simulink model "Sensorless_Fault_Tolerant_Control_IM_2"  (R2024a)
settings: Solver=VariableStepAuto  StartTime=0.0  StopTime=2  RelTol=1e-3
values from neighbouring files (symbols this model uses):
  Lm = 0.135    [Step_3_SVPWM.m]    (also in Step_With_MRAS_2c.m = 0.0055; Will_Check_3_Hk_2.m = 0.2)
  Ts = 1e-4    (= 0.0001)    [Step_3_SVPWM.m]    (also in Step_With_MRAS_2c.m; Will_Check_3_Hk_2.m)
undefined symbols (not defined in the file or in its folder): DiscIntNeverNeededParam, Ki, Kp, Param_Limit, R, S, Zp
libraries: spsACVoltageSourceLib x3, slpidlib x3, spsUniversalBridgeLib x3, spsCurrentMeasurementLib x3, spsVoltageMeasurementLib x3, spsAsynchronousMachineSIUnitsLib x2, spsDCVoltageSourceLib x1, spsAlphaBetaZerotodq0Lib x1, spsSVPWMGenerator2LevelLib x1, spsabctoAlphaBetaZeroLib x1, spsdq0toAlphaBetaZeroLib x1, spsGroundLib x1
settings Model: Creator=hkurt  LastModifiedBy=hkurt
settings RTWCC: GPUComputeCapability=3.5

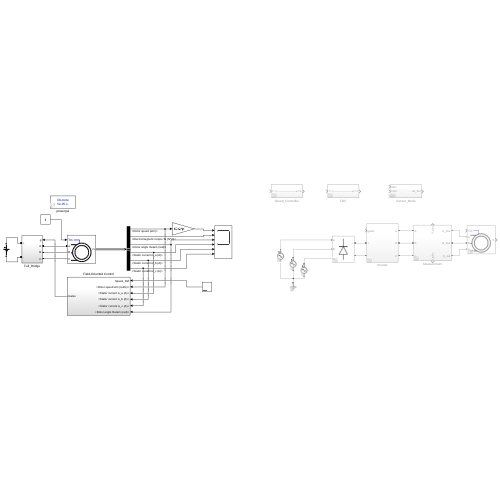
[thumbnail: Simulink's stored preview of the top-level diagram]
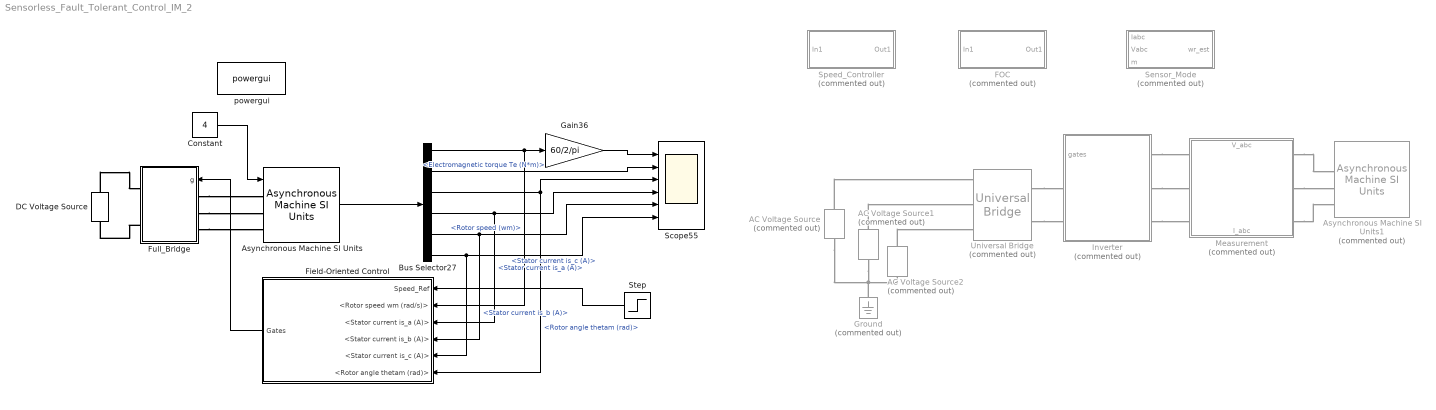
== system Sensorless_Fault_Tolerant_Control_IM_2 ==
  AC Voltage Source : spsACVoltageSourceLib/AC Voltage Source  Commented=on  Amplitude=400/sqrt(3)*sqrt(2)  Phase=0  Frequency=50  SampleTime=0  Measurements=None  BusType=swing  Pref=10e3  Qref=0  Qmin=-inf  Qmax=+inf
  AC Voltage Source1 : spsACVoltageSourceLib/AC Voltage Source  Commented=on  Amplitude=400/sqrt(3)*sqrt(2)  Phase=-120  Frequency=50  SampleTime=0  Measurements=None  BusType=swing  Pref=10e3  Qref=0  Qmin=-inf  Qmax=+inf
  AC Voltage Source2 : spsACVoltageSourceLib/AC Voltage Source  Commented=on  Amplitude=400/sqrt(3)*sqrt(2)  Phase=120  Frequency=50  SampleTime=0  Measurements=None  BusType=swing  Pref=10e3  Qref=0  Qmin=-inf  Qmax=+inf
  Asynchronous Machine SI Units : spsAsynchronousMachineSIUnitsLib/Asynchronous Machine SI Units  RotorType=Squirrel-cage  PresetModel="15:  5.4 HP (4KW)   400 V  50Hz 1430 RPM"  MechanicalLoad=Torque Tm  ShowDetailedParameters=on  ReferenceFrame=Rotor  Units=SI  MeasurementBus=off  NominalParameters=[4000 400 50]  VoltageRatio=1  Stator=[1.405 0.005839]  Rotor=[1.395 0.005839]  Cage1=[0.4155 0.002066]  Cage2=[0.4168 0.0003495]  Lm=0.1722  Mechanical=[0.0131 0.002985 2]  PolePairs=2  InitialConditions=[0 0 0 0 0 0 0 0]  SimulateSaturation=off  Saturation=[14.03593122, 27.81365428, 53.79336849, 72.68890987, 97.98006896, 148.6815601, 215.7428561, 302.9841135, 428.7778367 ; 230, 322, 414, 460, 506, 552, 598, 644, 690]  LoadFlowParameters=1492000  TsPowergui=0  TsBlock=-1  IterativeModel=Trapezoidal non iterative  IterativeDiscreteModel=Trapezoidal non iterative  Pmec=1.492e+006
  Asynchronous Machine SI Units1 : spsAsynchronousMachineSIUnitsLib/Asynchronous Machine SI Units  Commented=on  RotorType=Squirrel-cage  PresetModel="15:  5.4 HP (4KW)   400 V  50Hz 1430 RPM"  MechanicalLoad=Torque Tm  ShowDetailedParameters=on  ReferenceFrame=Rotor  Units=SI  MeasurementBus=off  NominalParameters=[4000 400 50]  VoltageRatio=1  Stator=[1.405 0.005839]  Rotor=[1.395 0.005839]  Cage1=[0.4155 0.002066]  Cage2=[0.4168 0.0003495]  Lm=0.1722  Mechanical=[0.0131 0.002985 2]  PolePairs=2  InitialConditions=[0 0 0 0 0 0 0 0]  SimulateSaturation=off  Saturation=[14.03593122, 27.81365428, 53.79336849, 72.68890987, 97.98006896, 148.6815601, 215.7428561, 302.9841135, 428.7778367 ; 230, 322, 414, 460, 506, 552, 598, 644, 690]  LoadFlowParameters=1492000  TsPowergui=0  TsBlock=-1  IterativeModel=Trapezoidal non iterative  IterativeDiscreteModel=Trapezoidal non iterative  Pmec=1.492e+006
  Bus Selector27 : BusSelector  OutputSignals=Mechanical.Rotor speed (wm),Mechanical.Electromagnetic torque Te (N*m),Mechanical.Rotor angle thetam (rad),Stator measurements.Stator current is_a (A),Stator measurements.Stator current is_b (A),Stator measurements.Stator current is_c (A)
  Constant : Constant  Value=4
  DC Voltage Source : spsDCVoltageSourceLib/DC Voltage Source  Amplitude=690  Measurements=None
  FOC : Subsystem  Commented=on
  Field-Oriented Control : Subsystem
  Full_Bridge : Subsystem
  Gain36 : Gain  Gain=60/2/pi
  Ground : spsGroundLib/Ground  Commented=on  LConnTagsString=a
  Inverter : Subsystem  Commented=on
  Measurement : Subsystem  Commented=on
      settings: PortSchema="{\"entries\":[{\"content\":{\"sides\":[{\"content\":{\"connectorIds\":[\"LConn1\",\"LConn2\",\"LConn3\"]},\"type\":\"ConnectorPlacement.EquallySpacedRectSide\",\"uuid\":\"2eb851a7-a296-4371-9492-5b9a24d98dc4\"},{\"content\":{\"connectorIds\":[\"RConn1\",\"RConn2\",\"RConn3\"],\"side\":\"RIGHT\"},\"type\":\"ConnectorPlacement.EquallySpacedRectSide\",\"uuid\":\"c9fabae8-70a9-40e0-bc91-dae6b4a86947\"},{\"content\":{\"connectorIds\":[\"Out2\"],\"side\":\"TOP\"},\"type\":\"ConnectorPlacement.EquallySpacedRectSide\",\"uuid\":\"f74854e5-c5df-4cc2-afef-707541dbedfe\"},{\"content\":{\"connectorIds\":[\"Out1\"],\"side\":\"BOTTOM\"},\"type\":\"ConnectorPlacement.EquallySpacedRectSide\",\"uuid\":\"696e7b86-8c4f-415d-8e64-0810cecd3876\"}]},\"type\":\"ConnectorPlacement.EquallySpacedConnector\",\"uuid\":\"1b4277bd-9dcb-424e-8124-b504b127c8b4\"}],\"packageUris\":[\"http://schema.mathworks.com/mf0/Connector/R2020b\"],\"version\":\"1.0\"}"
  Scope55 : Scope  NumInputPorts=6
  Sensor_Mode : Subsystem  Commented=on
  Speed_Controller : Subsystem  Commented=on
  Step : Step  Time=0.5  After=1200  SampleTime=0
  Universal Bridge : spsUniversalBridgeLib/Universal Bridge  Commented=on  Arms=3  SnubberResistance=1e5  SnubberCapacitance=inf  Device=Diodes  Ron=1e-3  Lon=0  ForwardVoltages="[  0  0  ]"  ForwardVoltage=0  GTOparameters=[ 10e-6 , 20e-6 ]  IGBTparameters=[ 1e-6 , 2e-6 ]  Measurements=None  Measurements_2=None  converterType=Rectifier
  powergui : sps_lib/powergui  Priority=1  SimulationMode=Discrete  SampleTime=50e-6  frequency=60  Iterations=50  frequencyindice=0  Pbase=100e6  ErrMax=1e-4  UnitsV=kV  UnitsW=MW  buscounter=0  FunctionMessages=off  echomessages=off  EnableUseOfTLC=off  CurrentSourceSwitches=off  DisableSnubberDevices=off  DisableRonSwitches=off  DisableVfSwitches=off  DisplayEquations=off  AutomaticDiscreteSolvers=off  SolverType=Tustin/Backward Euler (TBE)  Interpol=off  ExternalGateDelay=off  methode=off  Ts=100  x0status=blocks  SPID=on  SwTol=0  HookPort=off  NonlinearTolerance=1e-4  nMaxIteration=100  ContinueOnMaxIteration=off  RestoreLinks=warning  ResistiveCurrentMeasurement=off  Frange=[0:2:500]  Ylog=off  Xlog=on  ShowGrid=off  save=off  variable=ZData  structure=0  ZoomFFT=off  StartTime=0.0  cycles=1  DisplayStyle=1  fundamental=60  FreqAxis=off  MaxFrequency=1000  frequencyindicesteady=1  RmsSteady=1  display=off
  wires:
  Field-Oriented Control/1(Gates) -> Full_Bridge/1(g)
  Asynchronous Machine SI Units/1 -> Bus Selector27/1
  Gain36/1 -> Scope55/1
  Bus Selector27/1 -> Gain36/1, Field-Oriented Control/2(<Rotor speed wm (rad/s)>)  "<Rotor speed (wm)>"
  Bus Selector27/2 -> Scope55/2  "<Electromagnetic torque Te (N*m)>"
  Bus Selector27/3 -> Field-Oriented Control/6(<Rotor angle thetam (rad)>), Scope55/3  "<Rotor angle thetam (rad)>"
  Bus Selector27/4 -> Scope55/4, Field-Oriented Control/3(<Stator current is_a (A)>)  "<Stator current is_a (A)>"
  Bus Selector27/5 -> Field-Oriented Control/4(<Stator current is_b (A)>), Scope55/5  "<Stator current is_b (A)>"
  Bus Selector27/6 -> Scope55/6, Field-Oriented Control/5(<Stator current is_c (A)>)  "<Stator current is_c (A)>"
  Constant/1 -> Asynchronous Machine SI Units/1
  Step/1 -> Field-Oriented Control/1(Speed_Ref)
  connections:
  Full_Bridge/LConn1 -- Asynchronous Machine SI Units/LConn1
  Full_Bridge/LConn2 -- Asynchronous Machine SI Units/LConn2
  Full_Bridge/LConn3 -- Asynchronous Machine SI Units/LConn3
  DC Voltage Source/RConn1 -- Full_Bridge/RConn1
  Full_Bridge/RConn2 -- DC Voltage Source/LConn1
  Measurement/RConn1 -- Asynchronous Machine SI Units1/LConn1
  Measurement/RConn2 -- Asynchronous Machine SI Units1/LConn2
  Measurement/RConn3 -- Asynchronous Machine SI Units1/LConn3
  Inverter/RConn1 -- Measurement/LConn1
  Inverter/RConn2 -- Measurement/LConn2
  Inverter/RConn3 -- Measurement/LConn3
  Universal Bridge/RConn1 -- Inverter/LConn1
  Universal Bridge/RConn2 -- Inverter/LConn2
  AC Voltage Source/RConn1 -- Universal Bridge/LConn1
  AC Voltage Source1/RConn1 -- Universal Bridge/LConn2
  AC Voltage Source2/RConn1 -- Universal Bridge/LConn3
  Ground/LConn1 -- AC Voltage Source1/LConn1 -- AC Voltage Source/LConn1 -- AC Voltage Source2/LConn1

== system Sensorless_Fault_Tolerant_Control_IM_2/FOC ==
  In1 : Inport
  Out1 : Outport
  wires:
  In1/1 -> Out1/1

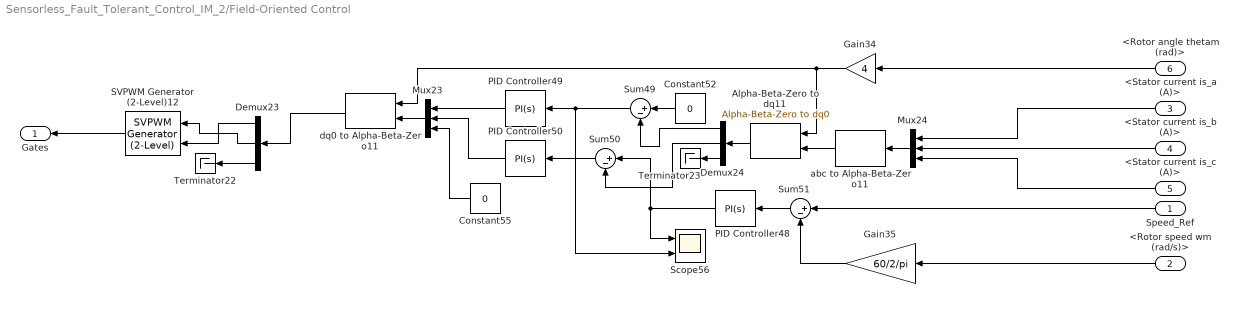
== system Sensorless_Fault_Tolerant_Control_IM_2/Field-Oriented Control ==
  Speed_Ref : Inport
  <Rotor speed wm (rad/s)> : Inport  Port=2
  <Stator current is_a (A)> : Inport  Port=3
  <Stator current is_b (A)> : Inport  Port=4
  <Stator current is_c (A)> : Inport  Port=5
  <Rotor angle thetam (rad)> : Inport  Port=6
  Alpha-Beta-Zero to dq11 : spsAlphaBetaZerotodq0Lib/Alpha-Beta-Zero to dq0  Alignment=90 degrees behind phase A axis
  Constant52 : Constant  Value=0
  Constant55 : Constant  Value=0
  Demux23 : Demux  Outputs=3
  Demux24 : Demux  Outputs=3
  Gain34 : Gain  Gain=4
  Gain35 : Gain  Gain=60/2/pi
  Mux23 : Mux  Inputs=3
  Mux24 : Mux  Inputs=3
  PID Controller48 : slpidlib/PID Controller  Controller=PI  Form=Parallel  TimeDomain=Continuous-time  UseExternalTs=off  SampleTime=-1  IntegratorMethod=Forward Euler  FilterMethod=Forward Euler  ControllerParametersSource=internal  P=0.5  I=10  UseKiTs=off  D=0  UseExternalDerivativeSource=off  N=100  UseFilter=on  TunerSelectOption=Transfer Function Based (PID Tuner App)  InitialConditionSource=internal  InitialConditionForIntegrator=0  InitialConditionForFilter=0  DifferentiatorICPrevScaledInput=0  ExternalReset=none  TrackingMode=off  Kt=1  LimitOutput=off  SatLimitsSource=internal  UpperSaturationLimit=inf  LowerSaturationLimit=-inf  LinearizeAsGain=on  AntiWindupMode=none  Kb=1  LimitIntegrator=off  UpperIntegratorSaturationLimit=inf  LowerIntegratorSaturationLimit=-inf  POutMin=[]  POutMax=[]  IOutMin=[]  IOutMax=[]  DOutMin=[]  DOutMax=[]  NOutMin=[]  NOutMax=[]  SumOutMin=[]  SumOutMax=[]  SaturationOutMin=[]  SaturationOutMax=[]  PParamMin=[]  PParamMax=[]  IParamMin=[]  IParamMax=[]  DParamMin=[]  DParamMax=[]  NParamMin=[]  NParamMax=[]  KbParamMin=[]  KbParamMax=[]  KtParamMin=[]  KtParamMax=[]  KbOutMin=[]  KbOutMax=[]  KtOutMin=[]  KtOutMax=[]  IntegratorOutMin=[]  IntegratorOutMax=[]  FilterOutMin=[]  FilterOutMax=[]  SumI1OutMin=[]  SumI1OutMax=[]  SumI2OutMin=[]  SumI2OutMax=[]  SumI3OutMin=[]  SumI3OutMax=[]  SumI4OutMin=[]  SumI4OutMax=[]  SumDOutMin=[]  SumDOutMax=[]  DifferentiatorOutMin=[]  DifferentiatorOutMax=[]  FilterDiffOutCoefMin=[]  FilterDiffOutCoefMax=[]  ReciprocalOutMin=[]  ReciprocalOutMax=[]  SumDenOutMin=[]  SumDenOutMax=[]  SumNumOutMin=[]  SumNumOutMax=[]  DivideOutMin=[]  DivideOutMax=[]  UdiffTsProdOutMin=[]  UdiffTsProdOutMax=[]  NTsProdOutMin=[]  NTsProdOutMax=[]  UintegralTsProdOutMin=[]  UintegralTsProdOutMax=[]  UngainTsProdOutMin=[]  UngainTsProdOutMax=[]  ClampingZeroOutDataTypeStr=Inherit: Inherit via back propagation  ClampingZeroOutMin=[]  ClampingZeroOutMax=[]  FilterDenConstantOutDataTypeStr=Inherit: Inherit via back propagation  FilterDenConstantOutMin=[]  FilterDenConstantOutMax=[]  PCopyOutDataTypeStr=Inherit: Inherit via back propagation  PCopyOutMin=[]  PCopyOutMax=[]  NCopyOutDataTypeStr=Inherit: Inherit via back propagation  NCopyOutMin=[]  NCopyOutMax=[]  IntegratorContinuousStateAttributes=''  IntegratorStateMustResolveToSignalObject=off  IntegratorRTWStateStorageClass=Auto  FilterContinuousStateAttributes=''  FilterStateMustResolveToSignalObject=off  FilterRTWStateStorageClass=Auto  ParallelPVariant=InternalParameters  IdealPVariant=Disabled  IVariant=InternalParameters  DVariant=Disabled  IntegratorVariant=Continuous  SatVariant=Disabled  AWVariant=Passthrough  PCopyVariant=Disabled  TRVariant=Disabled  FdbkBlocksVariant=Forward  IdealPFdbkVariant=Disabled  SatFdbkVariant=Disabled  DerivativeFilterVariant=Disabled  NVariant=Disabled  NCopyVariant=Disabled_SignalSpec  FilterICVariant=Disabled  IntegratorICVariant=InternalICs  ExternalResetVariant=Disabled  TRSumVariant=Passthrough  SumFdbkVariant=Disabled  SumVariant=Sum_PI  TsampFilterVariant=InternalTs  TsampNgainVariant=Passthrough  TsampIntegralVariant=Disabled_SignalSpec  ExternalSaturationOutDataTypeStr=Inherit: Same as second input  DerivativeSourceVariant=Disabled
  PID Controller49 : slpidlib/PID Controller  Controller=PI  Form=Parallel  TimeDomain=Continuous-time  UseExternalTs=off  SampleTime=-1  IntegratorMethod=Forward Euler  FilterMethod=Forward Euler  ControllerParametersSource=internal  P=10  I=2000  UseKiTs=off  D=0  UseExternalDerivativeSource=off  N=100  UseFilter=on  TunerSelectOption=Transfer Function Based (PID Tuner App)  InitialConditionSource=internal  InitialConditionForIntegrator=0  InitialConditionForFilter=0  DifferentiatorICPrevScaledInput=0  ExternalReset=none  TrackingMode=off  Kt=1  LimitOutput=off  SatLimitsSource=internal  UpperSaturationLimit=inf  LowerSaturationLimit=-inf  LinearizeAsGain=on  AntiWindupMode=none  Kb=1  LimitIntegrator=off  UpperIntegratorSaturationLimit=inf  LowerIntegratorSaturationLimit=-inf  POutMin=[]  POutMax=[]  IOutMin=[]  IOutMax=[]  DOutMin=[]  DOutMax=[]  NOutMin=[]  NOutMax=[]  SumOutMin=[]  SumOutMax=[]  SaturationOutMin=[]  SaturationOutMax=[]  PParamMin=[]  PParamMax=[]  IParamMin=[]  IParamMax=[]  DParamMin=[]  DParamMax=[]  NParamMin=[]  NParamMax=[]  KbParamMin=[]  KbParamMax=[]  KtParamMin=[]  KtParamMax=[]  KbOutMin=[]  KbOutMax=[]  KtOutMin=[]  KtOutMax=[]  IntegratorOutMin=[]  IntegratorOutMax=[]  FilterOutMin=[]  FilterOutMax=[]  SumI1OutMin=[]  SumI1OutMax=[]  SumI2OutMin=[]  SumI2OutMax=[]  SumI3OutMin=[]  SumI3OutMax=[]  SumI4OutMin=[]  SumI4OutMax=[]  SumDOutMin=[]  SumDOutMax=[]  DifferentiatorOutMin=[]  DifferentiatorOutMax=[]  FilterDiffOutCoefMin=[]  FilterDiffOutCoefMax=[]  ReciprocalOutMin=[]  ReciprocalOutMax=[]  SumDenOutMin=[]  SumDenOutMax=[]  SumNumOutMin=[]  SumNumOutMax=[]  DivideOutMin=[]  DivideOutMax=[]  UdiffTsProdOutMin=[]  UdiffTsProdOutMax=[]  NTsProdOutMin=[]  NTsProdOutMax=[]  UintegralTsProdOutMin=[]  UintegralTsProdOutMax=[]  UngainTsProdOutMin=[]  UngainTsProdOutMax=[]  ClampingZeroOutDataTypeStr=Inherit: Inherit via back propagation  ClampingZeroOutMin=[]  ClampingZeroOutMax=[]  FilterDenConstantOutDataTypeStr=Inherit: Inherit via back propagation  FilterDenConstantOutMin=[]  FilterDenConstantOutMax=[]  PCopyOutDataTypeStr=Inherit: Inherit via back propagation  PCopyOutMin=[]  PCopyOutMax=[]  NCopyOutDataTypeStr=Inherit: Inherit via back propagation  NCopyOutMin=[]  NCopyOutMax=[]  IntegratorContinuousStateAttributes=''  IntegratorStateMustResolveToSignalObject=off  IntegratorRTWStateStorageClass=Auto  FilterContinuousStateAttributes=''  FilterStateMustResolveToSignalObject=off  FilterRTWStateStorageClass=Auto  ParallelPVariant=InternalParameters  IdealPVariant=Disabled  IVariant=InternalParameters  DVariant=Disabled  IntegratorVariant=Continuous  SatVariant=Disabled  AWVariant=Passthrough  PCopyVariant=Disabled  TRVariant=Disabled  FdbkBlocksVariant=Forward  IdealPFdbkVariant=Disabled  SatFdbkVariant=Disabled  DerivativeFilterVariant=Disabled  NVariant=Disabled  NCopyVariant=Disabled_SignalSpec  FilterICVariant=Disabled  IntegratorICVariant=InternalICs  ExternalResetVariant=Disabled  TRSumVariant=Passthrough  SumFdbkVariant=Disabled  SumVariant=Sum_PI  TsampFilterVariant=InternalTs  TsampNgainVariant=Passthrough  TsampIntegralVariant=Disabled_SignalSpec  ExternalSaturationOutDataTypeStr=Inherit: Same as second input  DerivativeSourceVariant=Disabled
  PID Controller50 : slpidlib/PID Controller  Controller=PI  Form=Parallel  TimeDomain=Continuous-time  UseExternalTs=off  SampleTime=-1  IntegratorMethod=Forward Euler  FilterMethod=Forward Euler  ControllerParametersSource=internal  P=10  I=2000  UseKiTs=off  D=0  UseExternalDerivativeSource=off  N=100  UseFilter=on  TunerSelectOption=Transfer Function Based (PID Tuner App)  InitialConditionSource=internal  InitialConditionForIntegrator=0  InitialConditionForFilter=0  DifferentiatorICPrevScaledInput=0  ExternalReset=none  TrackingMode=off  Kt=1  LimitOutput=off  SatLimitsSource=internal  UpperSaturationLimit=inf  LowerSaturationLimit=-inf  LinearizeAsGain=on  AntiWindupMode=none  Kb=1  LimitIntegrator=off  UpperIntegratorSaturationLimit=inf  LowerIntegratorSaturationLimit=-inf  POutMin=[]  POutMax=[]  IOutMin=[]  IOutMax=[]  DOutMin=[]  DOutMax=[]  NOutMin=[]  NOutMax=[]  SumOutMin=[]  SumOutMax=[]  SaturationOutMin=[]  SaturationOutMax=[]  PParamMin=[]  PParamMax=[]  IParamMin=[]  IParamMax=[]  DParamMin=[]  DParamMax=[]  NParamMin=[]  NParamMax=[]  KbParamMin=[]  KbParamMax=[]  KtParamMin=[]  KtParamMax=[]  KbOutMin=[]  KbOutMax=[]  KtOutMin=[]  KtOutMax=[]  IntegratorOutMin=[]  IntegratorOutMax=[]  FilterOutMin=[]  FilterOutMax=[]  SumI1OutMin=[]  SumI1OutMax=[]  SumI2OutMin=[]  SumI2OutMax=[]  SumI3OutMin=[]  SumI3OutMax=[]  SumI4OutMin=[]  SumI4OutMax=[]  SumDOutMin=[]  SumDOutMax=[]  DifferentiatorOutMin=[]  DifferentiatorOutMax=[]  FilterDiffOutCoefMin=[]  FilterDiffOutCoefMax=[]  ReciprocalOutMin=[]  ReciprocalOutMax=[]  SumDenOutMin=[]  SumDenOutMax=[]  SumNumOutMin=[]  SumNumOutMax=[]  DivideOutMin=[]  DivideOutMax=[]  UdiffTsProdOutMin=[]  UdiffTsProdOutMax=[]  NTsProdOutMin=[]  NTsProdOutMax=[]  UintegralTsProdOutMin=[]  UintegralTsProdOutMax=[]  UngainTsProdOutMin=[]  UngainTsProdOutMax=[]  ClampingZeroOutDataTypeStr=Inherit: Inherit via back propagation  ClampingZeroOutMin=[]  ClampingZeroOutMax=[]  FilterDenConstantOutDataTypeStr=Inherit: Inherit via back propagation  FilterDenConstantOutMin=[]  FilterDenConstantOutMax=[]  PCopyOutDataTypeStr=Inherit: Inherit via back propagation  PCopyOutMin=[]  PCopyOutMax=[]  NCopyOutDataTypeStr=Inherit: Inherit via back propagation  NCopyOutMin=[]  NCopyOutMax=[]  IntegratorContinuousStateAttributes=''  IntegratorStateMustResolveToSignalObject=off  IntegratorRTWStateStorageClass=Auto  FilterContinuousStateAttributes=''  FilterStateMustResolveToSignalObject=off  FilterRTWStateStorageClass=Auto  ParallelPVariant=InternalParameters  IdealPVariant=Disabled  IVariant=InternalParameters  DVariant=Disabled  IntegratorVariant=Continuous  SatVariant=Disabled  AWVariant=Passthrough  PCopyVariant=Disabled  TRVariant=Disabled  FdbkBlocksVariant=Forward  IdealPFdbkVariant=Disabled  SatFdbkVariant=Disabled  DerivativeFilterVariant=Disabled  NVariant=Disabled  NCopyVariant=Disabled_SignalSpec  FilterICVariant=Disabled  IntegratorICVariant=InternalICs  ExternalResetVariant=Disabled  TRSumVariant=Passthrough  SumFdbkVariant=Disabled  SumVariant=Sum_PI  TsampFilterVariant=InternalTs  TsampNgainVariant=Passthrough  TsampIntegralVariant=Disabled_SignalSpec  ExternalSaturationOutDataTypeStr=Inherit: Same as second input  DerivativeSourceVariant=Disabled
  SVPWM Generator (2-Level)12 : spsSVPWMGenerator2LevelLib/SVPWM Generator (2-Level)  InputType=alpha-beta components  SwitchingPattern=Pattern #1  Fc=5000  ParUref=[0.8 -30 50]  Ts=0
  Scope56 : Scope  NumInputPorts=2
  Sum49 : Sum  Inputs=|+-
  Sum50 : Sum  Inputs=|+-
  Sum51 : Sum  Inputs=|+-
  Terminator22 : Terminator
  Terminator23 : Terminator
  abc to Alpha-Beta-Zero11 : spsabctoAlphaBetaZeroLib/abc to Alpha-Beta-Zero
  dq0 to Alpha-Beta-Zero11 : spsdq0toAlphaBetaZeroLib/dq0 to Alpha-Beta-Zero  Alignment=90 degrees behind phase A axis
  Gates : Outport
  wires:
  <Rotor angle thetam (rad)>/1 -> Gain34/1
  Mux23/1 -> dq0 to Alpha-Beta-Zero11/1
  Demux24/3 -> Terminator23/1
  Alpha-Beta-Zero to dq11/1 -> Demux24/1
  Constant55/1 -> Mux23/3
  Demux24/2 -> Sum50/2
  Mux24/1 -> abc to Alpha-Beta-Zero11/1
  <Rotor speed wm (rad/s)>/1 -> Gain35/1
  Constant52/1 -> Sum49/1
  Sum51/1 -> PID Controller48/1
  Gain34/1 -> Alpha-Beta-Zero to dq11/2, dq0 to Alpha-Beta-Zero11/2
  Gain35/1 -> Sum51/2
  PID Controller49/1 -> Mux23/1
  SVPWM Generator (2-Level)12/1 -> Gates/1
  abc to Alpha-Beta-Zero11/1 -> Alpha-Beta-Zero to dq11/1
  <Stator current is_a (A)>/1 -> Mux24/1
  <Stator current is_c (A)>/1 -> Mux24/3
  PID Controller50/1 -> Mux23/2
  dq0 to Alpha-Beta-Zero11/1 -> Demux23/1
  <Stator current is_b (A)>/1 -> Mux24/2
  Demux23/1 -> SVPWM Generator (2-Level)12/1
  Sum49/1 -> Scope56/2, PID Controller49/1
  Demux24/1 -> Sum49/2
  Demux23/2 -> SVPWM Generator (2-Level)12/2
  Speed_Ref/1 -> Sum51/1
  Demux23/3 -> Terminator22/1
  Sum50/1 -> PID Controller50/1
  PID Controller48/1 -> Scope56/1, Sum50/1

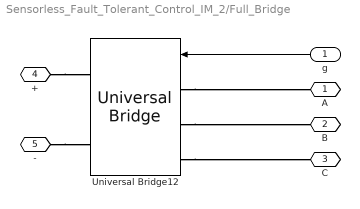
== system Sensorless_Fault_Tolerant_Control_IM_2/Full_Bridge ==
  g : Inport
  Universal Bridge12 : spsUniversalBridgeLib/Universal Bridge  Arms=3  SnubberResistance=1e5  SnubberCapacitance=inf  Device=IGBT / Diodes  Ron=1e-3  Lon=0  ForwardVoltages="[  0  0  ]"  ForwardVoltage=0  GTOparameters=[ 10e-6 , 20e-6 ]  IGBTparameters=[ 1e-6 , 2e-6 ]  Measurements=None  Measurements_2=None  converterType=Rectifier
  A : PMIOPort  Side=Left
  B : PMIOPort  Port=2  Side=Left
  C : PMIOPort  Port=3  Side=Left
  + : PMIOPort  Port=4  Side=Right
  - : PMIOPort  Port=5  Side=Right
  wires:
  g/1 -> Universal Bridge12/1
  connections:
  Universal Bridge12/LConn1 -- A/RConn1
  +/RConn1 -- Universal Bridge12/RConn1
  Universal Bridge12/LConn2 -- B/RConn1
  Universal Bridge12/LConn3 -- C/RConn1
  -/RConn1 -- Universal Bridge12/RConn2

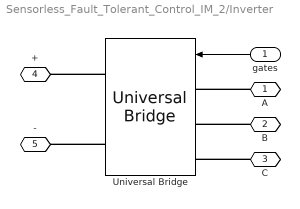
== system Sensorless_Fault_Tolerant_Control_IM_2/Inverter ==
  gates : Inport
  Universal Bridge : spsUniversalBridgeLib/Universal Bridge  Arms=3  SnubberResistance=1e5  SnubberCapacitance=inf  Device=IGBT / Diodes  Ron=1e-3  Lon=0  ForwardVoltages="[  0  0  ]"  ForwardVoltage=0  GTOparameters=[ 10e-6 , 20e-6 ]  IGBTparameters=[ 1e-6 , 2e-6 ]  Measurements=None  Measurements_2=None  converterType=Rectifier
  A : PMIOPort  Side=Right
  B : PMIOPort  Port=2  Side=Right
  C : PMIOPort  Port=3  Side=Right
  + : PMIOPort  Port=4  Side=Left
  - : PMIOPort  Port=5  Side=Left
  wires:
  gates/1 -> Universal Bridge/1
  connections:
  Universal Bridge/RConn1 -- +/RConn1
  Universal Bridge/RConn2 -- -/RConn1
  A/RConn1 -- Universal Bridge/LConn1
  B/RConn1 -- Universal Bridge/LConn2
  C/RConn1 -- Universal Bridge/LConn3

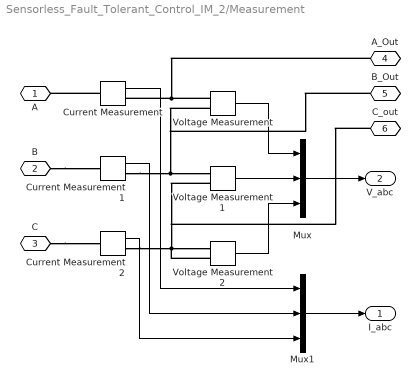
== system Sensorless_Fault_Tolerant_Control_IM_2/Measurement ==
  Current Measurement : spsCurrentMeasurementLib/Current Measurement  PhasorSimulation=off  OutputType=Complex  PSBequivalent=0
  Current Measurement1 : spsCurrentMeasurementLib/Current Measurement  PhasorSimulation=off  OutputType=Complex  PSBequivalent=0
  Current Measurement2 : spsCurrentMeasurementLib/Current Measurement  PhasorSimulation=off  OutputType=Complex  PSBequivalent=0
  Mux : Mux  Inputs=3
  Mux1 : Mux  Inputs=3
  Voltage Measurement : spsVoltageMeasurementLib/Voltage Measurement  PhasorSimulation=off  OutputType=Complex  PSBequivalent=0
  Voltage Measurement1 : spsVoltageMeasurementLib/Voltage Measurement  PhasorSimulation=off  OutputType=Complex  PSBequivalent=0
  Voltage Measurement2 : spsVoltageMeasurementLib/Voltage Measurement  PhasorSimulation=off  OutputType=Complex  PSBequivalent=0
  A : PMIOPort  Side=Left
  B : PMIOPort  Port=2  Side=Left
  C : PMIOPort  Port=3  Side=Left
  A_Out : PMIOPort  Port=4  Side=Right
  B_Out : PMIOPort  Port=5  Side=Right
  C_out : PMIOPort  Port=6  Side=Right
  I_abc : Outport
  V_abc : Outport  Port=2
  wires:
  Voltage Measurement1/1 -> Mux/2
  Voltage Measurement/1 -> Mux/1
  Voltage Measurement2/1 -> Mux/3
  Current Measurement/1 -> Mux1/1
  Current Measurement1/1 -> Mux1/2
  Current Measurement2/1 -> Mux1/3
  Mux/1 -> V_abc/1
  Mux1/1 -> I_abc/1
  connections:
  Voltage Measurement/LConn1 -- A_Out/RConn1 -- Current Measurement/RConn1
  Current Measurement1/RConn1 -- B_Out/RConn1 -- Voltage Measurement/LConn2 -- Voltage Measurement1/LConn1
  Current Measurement2/RConn1 -- Voltage Measurement1/LConn2 -- C_out/RConn1 -- Voltage Measurement2/LConn2 -- Voltage Measurement2/LConn1
  Current Measurement/LConn1 -- A/RConn1
  B/RConn1 -- Current Measurement1/LConn1
  C/RConn1 -- Current Measurement2/LConn1

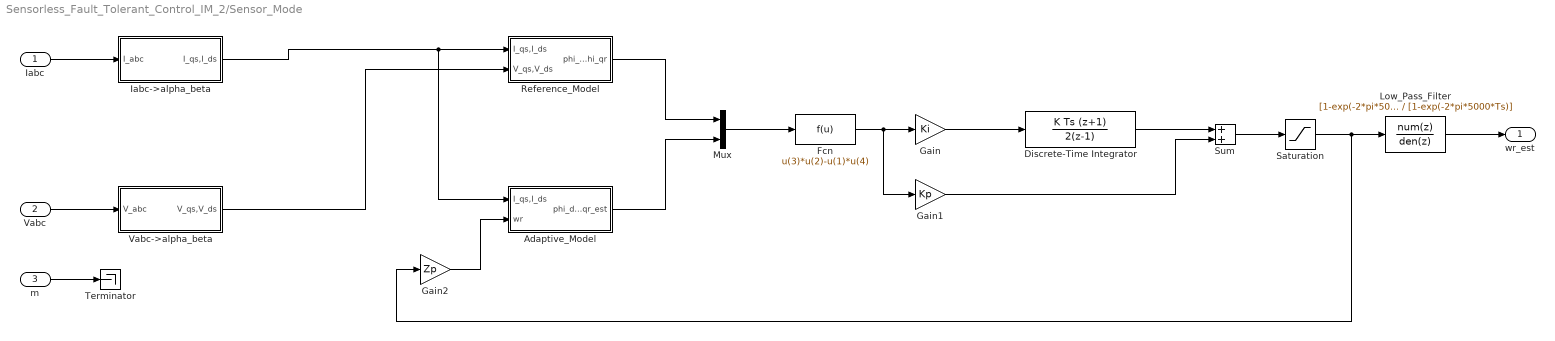
== system Sensorless_Fault_Tolerant_Control_IM_2/Sensor_Mode ==
  Iabc : Inport
  Vabc : Inport  Port=2
  m : Inport  Port=3
  Adaptive_Model : Subsystem
  Discrete-Time Integrator : DiscreteIntegrator  IntegratorMethod=Integration: Trapezoidal  SampleTime=Ts  LimitOutput=on  UpperSaturationLimit=Param_Limit(1)  LowerSaturationLimit=Param_Limit(2)  ICPrevOutput=DiscIntNeverNeededParam  ICPrevScaledInput=DiscIntNeverNeededParam
  Fcn : Fcn  Expr=u(3)*u(2)-u(1)*u(4)
  Gain : Gain  Gain=Ki
  Gain1 : Gain  Gain=Kp
  Gain2 : Gain  Gain=Zp
  Iabc->alpha_beta : Subsystem
  Low_Pass_Filter : DiscreteTransferFcn  Numerator=[1-exp(-2*pi*5000*Ts)]  Denominator=[1-exp(-2*pi*5000*Ts)]
  Mux : Mux  Inputs=2
  Reference_Model : Subsystem
  Saturation : Saturate  UpperLimit=Param_Limit(1)  LowerLimit=Param_Limit(1)
  Sum : Sum
  Terminator : Terminator
  Vabc->alpha_beta : Subsystem
  wr_est : Outport
  wires:
  Iabc/1 -> Iabc->alpha_beta/1(I_abc)
  Vabc->alpha_beta/1(V_qs,V_ds) -> Reference_Model/2(V_qs,V_ds)
  Vabc/1 -> Vabc->alpha_beta/1(V_abc)
  Iabc->alpha_beta/1(I_qs,I_ds) -> Adaptive_Model/1(I_qs,I_ds), Reference_Model/1(I_qs,I_ds)
  Reference_Model/1(phi_dr,phi_qr) -> Mux/1
  Adaptive_Model/1(phi_dr_est,phi_qr_est) -> Mux/2
  Mux/1 -> Fcn/1
  Fcn/1 -> Gain1/1, Gain/1
  Gain/1 -> Discrete-Time Integrator/1
  Discrete-Time Integrator/1 -> Sum/1
  Gain1/1 -> Sum/2
  Sum/1 -> Saturation/1
  Saturation/1 -> Gain2/1, Low_Pass_Filter/1
  Gain2/1 -> Adaptive_Model/2(wr)
  Low_Pass_Filter/1 -> wr_est/1
  m/1 -> Terminator/1

== system Sensorless_Fault_Tolerant_Control_IM_2/Speed_Controller ==
  In1 : Inport
  Out1 : Outport
  wires:
  In1/1 -> Out1/1

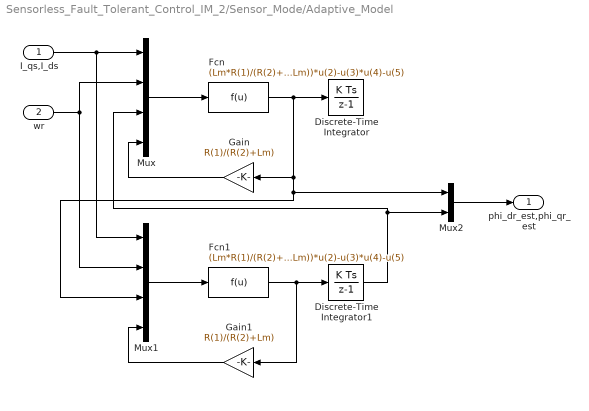
== system Sensorless_Fault_Tolerant_Control_IM_2/Sensor_Mode/Adaptive_Model ==
  I_qs,I_ds : Inport
  wr : Inport  Port=2
  Discrete-Time Integrator : DiscreteIntegrator  SampleTime=Ts  ICPrevOutput=DiscIntNeverNeededParam  ICPrevScaledInput=DiscIntNeverNeededParam
  Discrete-Time Integrator1 : DiscreteIntegrator  SampleTime=Ts  ICPrevOutput=DiscIntNeverNeededParam  ICPrevScaledInput=DiscIntNeverNeededParam
  Fcn : Fcn  Expr=(Lm*R(1)/(R(2)+Lm))*u(2)-u(3)*u(4)-u(5)
  Fcn1 : Fcn  Expr=(Lm*R(1)/(R(2)+Lm))*u(2)-u(3)*u(4)-u(5)
  Gain : Gain  Gain=R(1)/(R(2)+Lm)
  Gain1 : Gain  Gain=R(1)/(R(2)+Lm)
  Mux : Mux
  Mux1 : Mux
  Mux2 : Mux  Inputs=2
  phi_dr_est,phi_qr_est : Outport
  wires:
  Mux/1 -> Fcn/1
  Fcn/1 -> Mux2/1, Mux1/3, Gain/1, Discrete-Time Integrator/1
  Gain/1 -> Mux/4
  wr/1 -> Mux/2, Mux1/2
  Mux1/1 -> Fcn1/1
  I_qs,I_ds/1 -> Mux1/1, Mux/1
  Gain1/1 -> Mux1/4
  Fcn1/1 -> Gain1/1, Discrete-Time Integrator1/1
  Discrete-Time Integrator1/1 -> Mux2/2, Mux/3
  Mux2/1 -> phi_dr_est,phi_qr_est/1

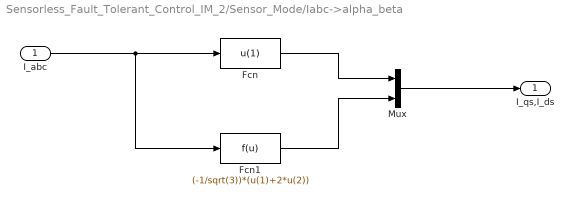
== system Sensorless_Fault_Tolerant_Control_IM_2/Sensor_Mode/Iabc->alpha_beta ==
  I_abc : Inport
  Fcn : Fcn  Expr=u(1)
  Fcn1 : Fcn  Expr=(-1/sqrt(3))*(u(1)+2*u(2))
  Mux : Mux  Inputs=2
  I_qs,I_ds : Outport
  wires:
  I_abc/1 -> Fcn/1, Fcn1/1
  Mux/1 -> I_qs,I_ds/1
  Fcn/1 -> Mux/1
  Fcn1/1 -> Mux/2

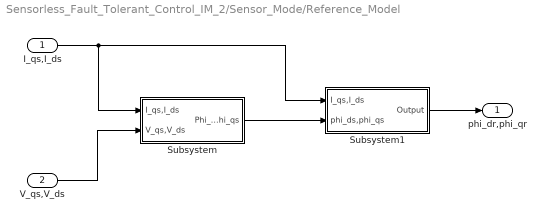
== system Sensorless_Fault_Tolerant_Control_IM_2/Sensor_Mode/Reference_Model ==
  I_qs,I_ds : Inport
  V_qs,V_ds : Inport  Port=2
  Subsystem : Subsystem
  Subsystem1 : Subsystem
  phi_dr,phi_qr : Outport
  wires:
  I_qs,I_ds/1 -> Subsystem1/1(I_qs,I_ds), Subsystem/1(I_qs,I_ds)
  V_qs,V_ds/1 -> Subsystem/2(V_qs,V_ds)
  Subsystem/1("Phi_ds, Phi_qs") -> Subsystem1/2(phi_ds,phi_qs)
  Subsystem1/1(Output) -> phi_dr,phi_qr/1

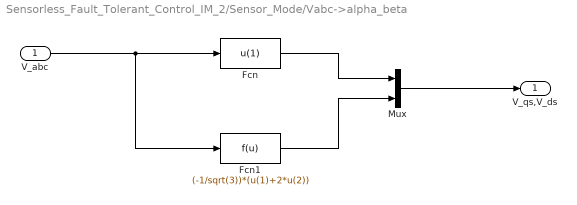
== system Sensorless_Fault_Tolerant_Control_IM_2/Sensor_Mode/Vabc->alpha_beta ==
  V_abc : Inport
  Fcn : Fcn  Expr=u(1)
  Fcn1 : Fcn  Expr=(-1/sqrt(3))*(u(1)+2*u(2))
  Mux : Mux  Inputs=2
  V_qs,V_ds : Outport
  wires:
  V_abc/1 -> Fcn/1, Fcn1/1
  Fcn/1 -> Mux/1
  Mux/1 -> V_qs,V_ds/1
  Fcn1/1 -> Mux/2

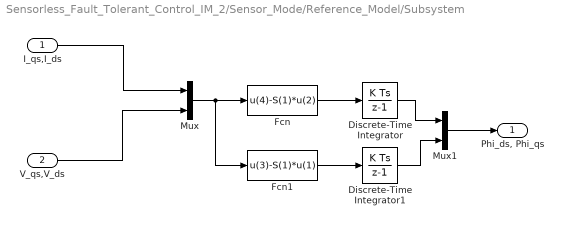
== system Sensorless_Fault_Tolerant_Control_IM_2/Sensor_Mode/Reference_Model/Subsystem ==
  I_qs,I_ds : Inport
  V_qs,V_ds : Inport  Port=2
  Discrete-Time Integrator : DiscreteIntegrator  SampleTime=1e-5  ICPrevOutput=DiscIntNeverNeededParam  ICPrevScaledInput=DiscIntNeverNeededParam
  Discrete-Time Integrator1 : DiscreteIntegrator  SampleTime=1e-5  ICPrevOutput=DiscIntNeverNeededParam  ICPrevScaledInput=DiscIntNeverNeededParam
  Fcn : Fcn  Expr=u(4)-S(1)*u(2)
  Fcn1 : Fcn  Expr=u(3)-S(1)*u(1)
  Mux : Mux  Inputs=2
  Mux1 : Mux  Inputs=2
  "Phi_ds, Phi_qs" : Outport
  wires:
  V_qs,V_ds/1 -> Mux/2
  I_qs,I_ds/1 -> Mux/1
  Fcn1/1 -> Discrete-Time Integrator1/1
  Mux/1 -> Fcn1/1, Fcn/1
  Fcn/1 -> Discrete-Time Integrator/1
  Discrete-Time Integrator/1 -> Mux1/1
  Discrete-Time Integrator1/1 -> Mux1/2
  Mux1/1 -> "Phi_ds, Phi_qs"/1

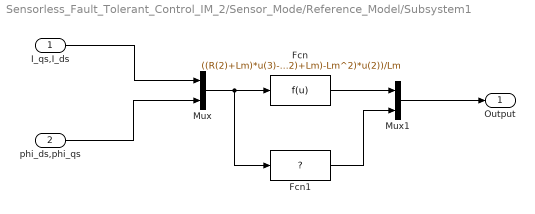
== system Sensorless_Fault_Tolerant_Control_IM_2/Sensor_Mode/Reference_Model/Subsystem1 ==
  I_qs,I_ds : Inport
  phi_ds,phi_qs : Inport  Port=2
  Fcn : Fcn  Expr=((R(2)+Lm)*u(3)-((S(2)+Lm)*(R(2)+Lm)-Lm^2)*u(2))/Lm
  Fcn1 : Fcn  Expr=?
  Mux : Mux  Inputs=2
  Mux1 : Mux  Inputs=2
  Output : Outport
  wires:
  I_qs,I_ds/1 -> Mux/1
  phi_ds,phi_qs/1 -> Mux/2
  Mux/1 -> Fcn1/1, Fcn/1
  Fcn/1 -> Mux1/1
  Fcn1/1 -> Mux1/2
  Mux1/1 -> Output/1
